simulink model "force_grav"  (R2021a)
settings: Solver=VariableStepAuto  StartTime=0.0  StopTime=100  RelTol=1e-3
values from neighbouring files (symbols this model uses):
  P = [real(P), imag(P)]    [black_pz.m]    (also in black_rlocus.m; black_rlocus_fine.m)
  R = rlocus(sys)    [black_rlocus.m]    (also in black_rlocus_fine.m = rlocus(sys,k))
undefined symbols (not defined in the file or in its folder): A_rocket, alpha_fine, Baro_exp, cm_fine, cm_lookup, Ct_rot, D, drag_lookup, drag_rot_lookup, drag_wave_lookup, g, h_0, I_s, I_x_lookup, I_yz_lookup, L_b, lift_lookup, lift_rot_lookup, m_burn, M_crit, M_fine, m_prop_max, m_wet, N, P_0, Phi, Psi, Q, r_E, S_e, T_b, T_lookup, T_max, T_max_s, t_P, t_S, Theta, U, V, W
libraries: simulink_extras x2
settings Model: Creator=EpEp  LastModifiedBy=EpEp
settings DebuggingCC: UnderSpecifiedDimensionMsg=warning

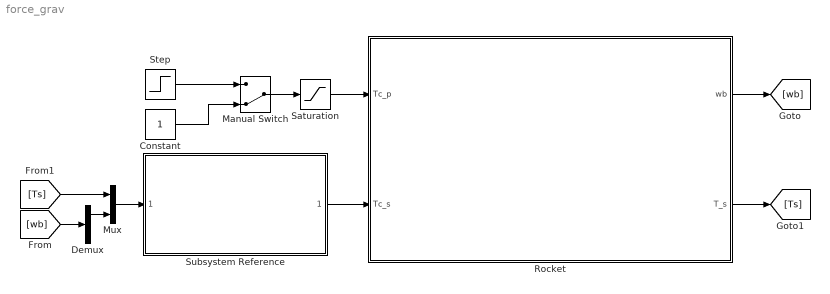
== system force_grav ==
  Constant : Constant
  Demux : Demux  Outputs=3
  Manual Switch : ManualSwitch  CurrentSetting=0
  Mux : Mux  Inputs=2
  Rocket : Subsystem
  Saturation : Saturate  UpperLimit=1  LowerLimit=0.5
  Step : Step  Time=10  Before=1  After=0  SampleTime=0
  Subsystem Reference : Subsystem  ReferencedSubsystem=roll_controller
  wires:
  Constant/1 -> Manual Switch/2
  Step/1 -> Manual Switch/1
  Manual Switch/1 -> Saturation/1
  Saturation/1 -> Rocket/1(Tc_p)
  Mux/1 -> Subsystem Reference/1
  Demux/1 -> Mux/2
  Subsystem Reference/1 -> Rocket/2(Tc_s)
  Rocket/1(wb) -> [wb]
  Rocket/2(T_s) -> [Ts]
  [wb] -> Demux/1
  [Ts] -> Mux/1

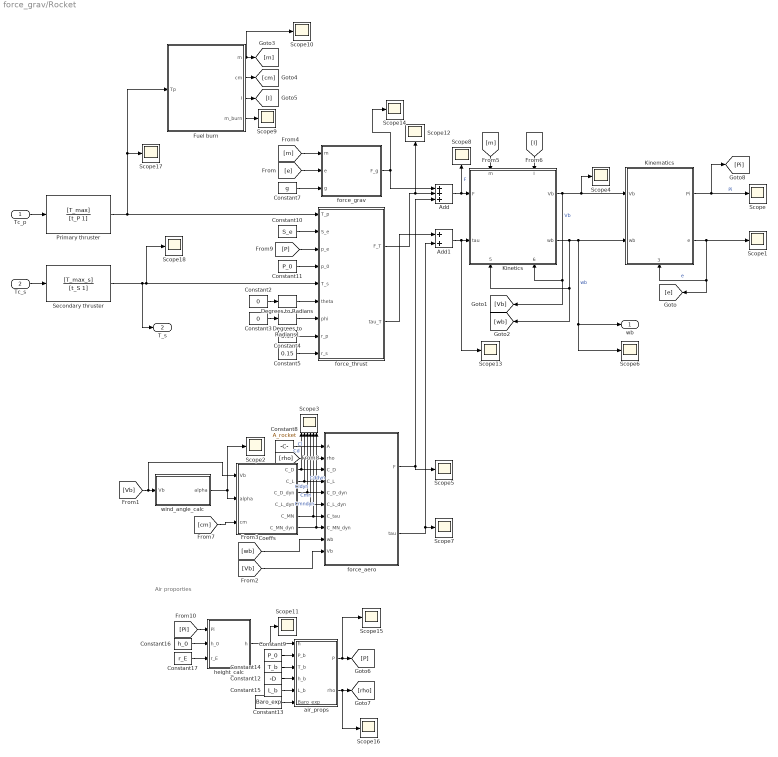
== system force_grav/Rocket ==
  note: Air proporties
  Tc_p : Inport
  Tc_s : Inport  Port=2
  Add : Sum  Inputs=+++
  Add1 : Sum
  Coeffs : Subsystem
  Constant10 : Constant  Value=S_e
  Constant11 : Constant  Value=P_0
  Constant12 : Constant  Value=-D
  Constant13 : Constant  Value=Baro_exp
  Constant14 : Constant  Value=T_b
  Constant15 : Constant  Value=L_b
  Constant16 : Constant  Value=h_0
  Constant17 : Constant  Value=r_E
  Constant2 : Constant  Value=0
  Constant3 : Constant  Value=0
  Constant4 : Constant  Value=0.55
  Constant5 : Constant  Value=0.15
  Constant7 : Constant  Value=g
  Constant8 : Constant  Value=A_rocket
  Constant9 : Constant  Value=P_0
  Degrees to Radians : simulink_extras/Transformations/Degrees to Radians
  Degrees to Radians1 : simulink_extras/Transformations/Degrees to Radians
  Fuel burn : Subsystem
  Kinematics : Subsystem
      settings: PortSchema="{\"entries\":[{\"content\":{\"sides\":[{\"content\":{\"connectorIds\":[\"In1\",\"In2\"]},\"type\":\"ConnectorPlacement.EquallySpacedRectSide\",\"uuid\":\"eae29983-0cae-4ee4-868d-1c50a6f3cfea\"},{\"content\":{\"connectorIds\":[\"Out1\",\"Out2\"],\"side\":\"RIGHT\"},\"type\":\"ConnectorPlacement.EquallySpacedRectSide\",\"uuid\":\"bdc65933-6547-4251-8b39-00a552207d7f\"},{\"content\":{\"connectorIds\":[],\"side\":\"TOP\"},\"type\":\"ConnectorPlacement.EquallySpacedRectSide\",\"uuid\":\"ee33c1e0-7d1f-4e43-84a0-58639e27ac5c\"},{\"content\":{\"connectorIds\":[\"In3\"],\"side\":\"BOTTOM\"},\"type\":\"ConnectorPlacement.EquallySpacedRectSide\",\"uuid\":\"b7ff67e5-658b-4688-8b54-a193f9f6d197\"}]},\"type\":\"ConnectorPlacement.EquallySpacedConnector\",\"uuid\":\"f4d120fb-b3cd-4fc8-b600-b4efda2a2057\"}],\"packageUris\":[\"http://schema.mathworks.com/mf0/Connector/R2020b\"],\"version\":\"1.0\"}"
  Kinetics : Subsystem
      settings: PortSchema="{\"entries\":[{\"content\":{\"sides\":[{\"content\":{\"connectorIds\":[\"In1\",\"In2\"]},\"type\":\"ConnectorPlacement.EquallySpacedRectSide\",\"uuid\":\"44e96cf1-b775-4685-9d80-77fe5197a3b8\"},{\"content\":{\"connectorIds\":[\"Out1\",\"Out2\"],\"side\":\"RIGHT\"},\"type\":\"ConnectorPlacement.EquallySpacedRectSide\",\"uuid\":\"1ce02f86-3039-4a72-8110-79d6c21885aa\"},{\"content\":{\"connectorIds\":[\"In3\",\"In4\"],\"side\":\"TOP\"},\"type\":\"ConnectorPlacement.EquallySpacedRectSide\",\"uuid\":\"c3c088af-4572-4447-8e34-ea7d8079d91e\"},{\"content\":{\"connectorIds\":[\"In5\",\"In6\"],\"side\":\"BOTTOM\"},\"type\":\"ConnectorPlacement.EquallySpacedRectSide\",\"uuid\":\"9c91a776-c86a-41f9-9dfe-00178419c6d9\"}]},\"type\":\"ConnectorPlacement.EquallySpacedConnector\",\"uuid\":\"6fbd1051-4f47-4787-a689-54b5a6d8998f\"}],\"packageUris\":[\"http://schema.mathworks.com/mf0/Connector/R2020b\"],\"version\":\"1.0\"}"
  Primary thruster : TransferFcn  Numerator=[T_max]  Denominator=[t_P 1]
  Scope{,1..2,4..18} (18 alike) : Scope
  Scope3 : Scope  NumInputPorts=6
  Secondary thruster : TransferFcn  Numerator=[T_max_s]  Denominator=[t_S 1]
  air_props : MATLAB Function  TreatAsAtomicUnit=on
  force_aero : MATLAB Function  TreatAsAtomicUnit=on
  force_grav : MATLAB Function  TreatAsAtomicUnit=on
  force_thrust : MATLAB Function  TreatAsAtomicUnit=on
  height_calc : MATLAB Function  TreatAsAtomicUnit=on
  wind_angle_calc : MATLAB Function  TreatAsAtomicUnit=on
  wb : Outport
  T_s : Outport  Port=2
  wires:
  Primary thruster/1 -> Fuel burn/1(Tp), Scope17/1, force_thrust/1(T_p)
  [Vb] -> Coeffs/1(Vb), wind_angle_calc/1(Vb)
  Fuel burn/1(m) -> Scope10/1, [m]
  Kinetics/2(wb) -> [wb], Kinetics/5(5), wb/1, Scope6/1, Kinematics/2(wb)  "wb"
  force_grav/1(F_g) -> Add/1, Scope14/1
  force_aero/2(tau) -> Add1/2, Scope7/1
  Kinematics/1(Pi) -> [Pi], Scope/1  "Pi"
  Kinematics/2(e) -> [e], Kinematics/3(3), Scope1/1  "e"
  Kinetics/1(Vb) -> [Vb], Kinetics/6(6), Scope4/1, Kinematics/1(Vb)  "Vb"
  air_props/2(rho) -> Scope16/1, [rho]
  Coeffs/3(C_D_dyn) -> Scope3/3, force_aero/5(C_D_dyn)  "Cddyn"
  height_calc/1(h) -> Scope11/1, air_props/1(h)
  Constant4/1 -> force_thrust/8(r_p)
  Constant3/1 -> Degrees to Radians1/1
  Add/1 -> Kinetics/1(F), Scope8/1  "F"
  Coeffs/2(C_L) -> Scope3/2, force_aero/4(C_L)  "Cl"
  Degrees to Radians1/1 -> force_thrust/7(phi)
  Add1/1 -> Scope13/1, Kinetics/2(tau)
  Coeffs/4(C_L_dyn) -> Scope3/4, force_aero/6(C_L_dyn)  "Cldyn"
  Coeffs/5(C_MN) -> Scope3/5, force_aero/7(C_tau)  "Cmn"
  Constant9/1 -> air_props/2(P_b)
  force_thrust/2(tau_T) -> Add1/1
  Coeffs/1(C_D) -> Scope3/1, force_aero/3(C_D)  "Cd"
  air_props/1(P) -> Scope15/1, [P]
  [Pi] -> height_calc/1(Pi)
  Constant14/1 -> air_props/3(T_b)
  Coeffs/6(C_MN_dyn) -> Scope3/6, force_aero/8(C_MN_dyn)  "Cmndyn"
  Constant5/1 -> force_thrust/9(r_s)
  Constant7/1 -> force_grav/3(g)
  wind_angle_calc/1(alpha) -> Scope2/1, Coeffs/2(alpha)
  [I] -> Kinetics/4(I)
  Constant16/1 -> height_calc/2(h_0)
  Constant11/1 -> force_thrust/4(p_0)
  Fuel burn/4(m_burn) -> Scope9/1
  [e] -> force_grav/2(e)
  Secondary thruster/1 -> T_s/1, Scope18/1, force_thrust/5(T_s)
  [m] -> force_grav/1(m)
  Constant2/1 -> Degrees to Radians/1
  Constant13/1 -> air_props/6(Baro_exp)
  [m] -> Kinetics/3(m)
  force_aero/1(F) -> Scope5/1, Add/3
  force_thrust/1(F_T) -> Add/2, Scope12/1
  Degrees to Radians/1 -> force_thrust/6(theta)
  [rho] -> force_aero/2(rho)
  [P] -> force_thrust/3(p_e)
  Constant12/1 -> air_props/4(h_b)
  Constant15/1 -> air_props/5(L_b)
  Constant8/1 -> force_aero/1(A)
  [wb] -> force_aero/9(wb)
  Constant10/1 -> force_thrust/2(S_e)
  Constant17/1 -> height_calc/3(r_E)
  Fuel burn/3(I) -> [I]
  [cm] -> Coeffs/3(cm)
  Fuel burn/2(cm) -> [cm]
  [Vb] -> force_aero/10(Vb)
  Tc_p/1 -> Primary thruster/1
  Tc_s/1 -> Secondary thruster/1

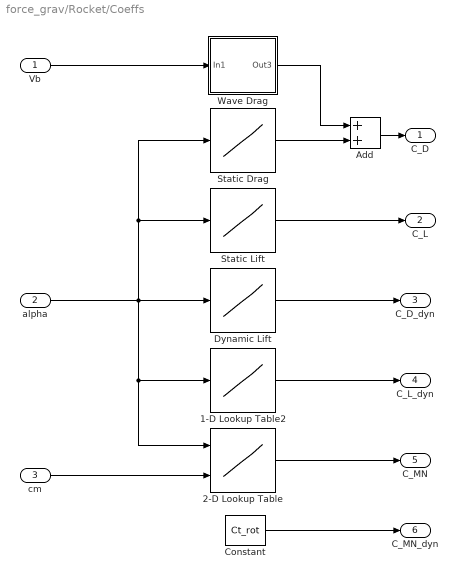
== system force_grav/Rocket/Coeffs ==
  Vb : Inport
  alpha : Inport  Port=2
  cm : Inport  Port=3
  1-D Lookup Table2 : Lookup_n-D  NumberOfTableDimensions=1  BreakpointsForDimension1=alpha_fine  Table=lift_rot_lookup  InternalRulePriority=Speed  RndMeth=Simplest  InputSameDT=on
  2-D Lookup Table : Lookup_n-D  BreakpointsForDimension1=alpha_fine  BreakpointsForDimension2=cm_fine  Table=T_lookup  InternalRulePriority=Speed  RndMeth=Simplest  InputSameDT=on
      settings: InputPortMap=u0,u1
  Add : Sum
  Constant : Constant  Value=Ct_rot
  Dynamic Lift : Lookup_n-D  NumberOfTableDimensions=1  BreakpointsForDimension1=alpha_fine  Table=drag_rot_lookup  InternalRulePriority=Speed  RndMeth=Simplest  InputSameDT=on
  Static Drag : Lookup_n-D  NumberOfTableDimensions=1  BreakpointsForDimension1=alpha_fine  Table=drag_lookup  InternalRulePriority=Speed  RndMeth=Simplest  InputSameDT=on
  Static Lift : Lookup_n-D  NumberOfTableDimensions=1  BreakpointsForDimension1=alpha_fine  Table=lift_lookup  InternalRulePriority=Speed  RndMeth=Simplest  InputSameDT=on
  Wave Drag : Subsystem
  C_D : Outport
  C_L : Outport  Port=2
  C_D_dyn : Outport  Port=3
  C_L_dyn : Outport  Port=4
  C_MN : Outport  Port=5
  C_MN_dyn : Outport  Port=6
  wires:
  alpha/1 -> Static Drag/1, Static Lift/1, 2-D Lookup Table/1, 1-D Lookup Table2/1, Dynamic Lift/1
  cm/1 -> 2-D Lookup Table/2
  Static Lift/1 -> C_L/1
  Dynamic Lift/1 -> C_D_dyn/1
  1-D Lookup Table2/1 -> C_L_dyn/1
  2-D Lookup Table/1 -> C_MN/1
  Constant/1 -> C_MN_dyn/1
  Static Drag/1 -> Add/2
  Vb/1 -> Wave Drag/1(In1)
  Wave Drag/1(Out3) -> Add/1
  Add/1 -> C_D/1

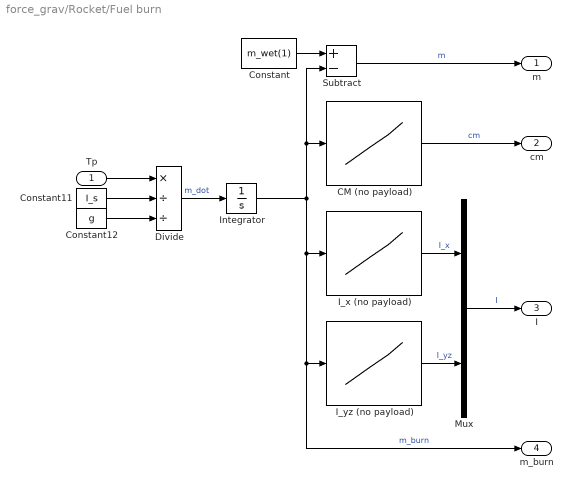
== system force_grav/Rocket/Fuel burn ==
  Tp : Inport
  CM (no payload) : Lookup_n-D  NumberOfTableDimensions=1  BreakpointsForDimension1=[0,m_prop_max*2]  Table=cm_lookup  InternalRulePriority=Speed  RndMeth=Simplest  InputSameDT=on
  Constant : Constant  Value=m_wet(1)
  Constant11 : Constant  Value=I_s
  Constant12 : Constant  Value=g
  Divide : Product  Inputs=*//
  I_x (no payload) : Lookup_n-D  NumberOfTableDimensions=1  BreakpointsForDimension1=[0,m_prop_max*2]  Table=I_x_lookup  InternalRulePriority=Speed  RndMeth=Simplest  InputSameDT=on
  I_yz (no payload) : Lookup_n-D  NumberOfTableDimensions=1  BreakpointsForDimension1=m_burn*2  Table=I_yz_lookup  InternalRulePriority=Speed  RndMeth=Simplest  InputSameDT=on
  Integrator : Integrator
  Mux : Mux  Inputs=2
  Subtract : Sum  Inputs=+-
  m : Outport
  cm : Outport  Port=2
  I : Outport  Port=3
  m_burn : Outport  Port=4
  wires:
  Divide/1 -> Integrator/1  "m_dot"
  Constant11/1 -> Divide/2
  Integrator/1 -> m_burn/1, I_yz (no payload)/1, I_x (no payload)/1, Subtract/2, CM (no payload)/1  "m_burn"
  Tp/1 -> Divide/1
  Constant/1 -> Subtract/1
  Subtract/1 -> m/1  "m"
  CM (no payload)/1 -> cm/1  "cm"
  I_x (no payload)/1 -> Mux/1  "I_x"
  I_yz (no payload)/1 -> Mux/2  "I_yz"
  Mux/1 -> I/1  "I"
  Constant12/1 -> Divide/3

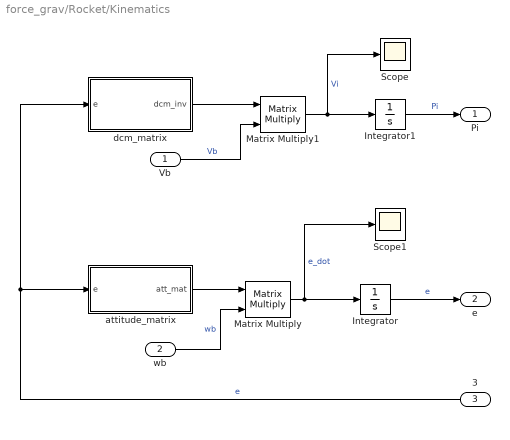
== system force_grav/Rocket/Kinematics ==
  Vb : Inport
  wb : Inport  Port=2
  3 : Inport  Port=3
  Integrator : Integrator  InitialCondition=[Phi;Theta;Psi]
  Integrator1 : Integrator  InitialCondition=[N;E;D]
  Matrix Multiply : Product  Multiplication=Matrix(*)
  Matrix Multiply1 : Product  Multiplication=Matrix(*)
  Scope : Scope
  Scope1 : Scope
  attitude_matrix : MATLAB Function  TreatAsAtomicUnit=on
  dcm_matrix : MATLAB Function  TreatAsAtomicUnit=on
  Pi : Outport
  e : Outport  Port=2
  wires:
  attitude_matrix/1(att_mat) -> Matrix Multiply/1
  wb/1 -> Matrix Multiply/2  "wb"
  Matrix Multiply/1 -> Scope1/1, Integrator/1  "e_dot"
  Integrator/1 -> e/1  "e"
  dcm_matrix/1(dcm_inv) -> Matrix Multiply1/1
  Vb/1 -> Matrix Multiply1/2  "Vb"
  Matrix Multiply1/1 -> Scope/1, Integrator1/1  "Vi"
  Integrator1/1 -> Pi/1  "Pi"
  3/1 -> dcm_matrix/1(e), attitude_matrix/1(e)  "e"

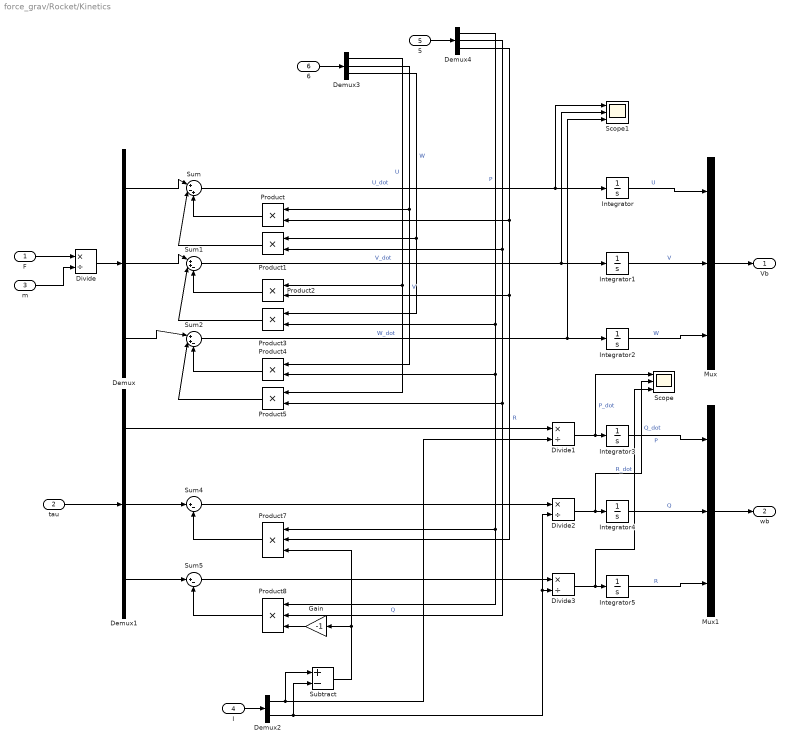
== system force_grav/Rocket/Kinetics ==
  F : Inport  PortDimensions=[3,1]
  tau : Inport  Port=2  PortDimensions=[3,1]
  m : Inport  Port=3
  I : Inport  Port=4
  5 : Inport  Port=5
  6 : Inport  Port=6
  Demux{,1,3..4} (4 alike) : Demux  Outputs=3
  Demux2 : Demux  Outputs=2
  Divide{,1..3} (4 alike) : Product  Inputs=*/
  Gain : Gain  Gain=-1
  Integrator : Integrator  InitialCondition=U
  Integrator1 : Integrator  InitialCondition=V
  Integrator2 : Integrator  InitialCondition=W
  Integrator3 : Integrator  InitialCondition=P
  Integrator4 : Integrator  InitialCondition=Q
  Integrator5 : Integrator  InitialCondition=R
  Mux : Mux  Inputs=3
  Mux1 : Mux  Inputs=3
  Product{,1..5} (6 alike) : Product
  Product7 : Product  Inputs=3
  Product8 : Product  Inputs=3
  Scope : Scope  NumInputPorts=3
  Scope1 : Scope  NumInputPorts=3
  Subtract : Sum  Inputs=+-
  Sum : Sum  Inputs=|+-+
  Sum1 : Sum  Inputs=|++-
  Sum2 : Sum  Inputs=|++-
  Sum4 : Sum  Inputs=|+-
  Sum5 : Sum  Inputs=|+-
  Vb : Outport  PortDimensions=[3,1]
  wb : Outport  Port=2  PortDimensions=[3,1]
  wires:
  Demux/1 -> Sum/1
  Demux1/3 -> Sum5/1
  Demux/2 -> Sum1/1
  Demux/3 -> Sum2/1
  Demux1/2 -> Sum4/1
  Product1/1 -> Sum/2
  Product/1 -> Sum/3
  Product3/1 -> Sum1/2
  Product2/1 -> Sum1/3
  Product4/1 -> Sum2/3
  Product5/1 -> Sum2/2
  F/1 -> Divide/1
  Divide/1 -> Demux/1
  m/1 -> Divide/2
  tau/1 -> Demux1/1
  Product7/1 -> Sum4/2
  Product8/1 -> Sum5/2
  Demux1/1 -> Divide1/1
  Divide1/1 -> Scope/1, Integrator3/1  "P_dot"
  Sum/1 -> Scope1/1, Integrator/1  "U_dot"
  Sum1/1 -> Scope1/2, Integrator1/1  "V_dot"
  Sum2/1 -> Scope1/3, Integrator2/1  "W_dot"
  I/1 -> Demux2/1
  Demux2/1 -> Divide1/2, Subtract/1
  Divide2/1 -> Scope/2, Integrator4/1  "Q_dot"
  Divide3/1 -> Scope/3, Integrator5/1  "R_dot"
  Sum5/1 -> Divide3/1
  Sum4/1 -> Divide2/1
  Demux2/2 -> Divide3/2, Divide2/2, Subtract/2
  Subtract/1 -> Product7/3, Gain/1
  Gain/1 -> Product8/3
  6/1 -> Demux3/1
  5/1 -> Demux4/1
  Demux3/2 -> Product4/1, Product/1  "V"
  Demux4/3 -> Product7/2, Product2/2, Product/2  "R"
  Demux3/3 -> Product3/1, Product1/1  "W"
  Demux4/1 -> Product3/2, Product8/1, Product7/1, Product4/2  "P"
  Demux3/1 -> Product5/1, Product2/1  "U"
  Demux4/2 -> Product1/2, Product5/2, Product8/2  "Q"
  Integrator/1 -> Mux/1  "U"
  Integrator2/1 -> Mux/3  "W"
  Integrator1/1 -> Mux/2  "V"
  Mux/1 -> Vb/1
  Integrator5/1 -> Mux1/3  "R"
  Integrator4/1 -> Mux1/2  "Q"
  Integrator3/1 -> Mux1/1  "P"
  Mux1/1 -> wb/1

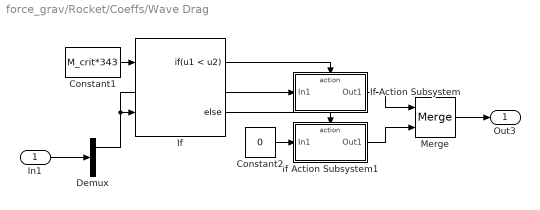
== system force_grav/Rocket/Coeffs/Wave Drag ==
  In1 : Inport
  Constant1 : Constant  Value=M_crit*343
  Constant2 : Constant  Value=0
  Demux : Demux  Outputs=3
  If : If  NumInputs=2  IfExpression=u1 < u2
  If Action Subsystem : Subsystem  TreatAsAtomicUnit=on
  If Action Subsystem1 : Subsystem  TreatAsAtomicUnit=on
  Merge : Merge
  Out3 : Outport
  wires:
  Merge/1 -> Out3/1
  If/2 -> If Action Subsystem1/Action
  Demux/1 -> If/2, If Action Subsystem/1(In1)
  If Action Subsystem1/1(Out1) -> Merge/2
  Constant1/1 -> If/1
  If Action Subsystem/1(Out1) -> Merge/1
  If/1 -> If Action Subsystem/Action
  Constant2/1 -> If Action Subsystem1/1(In1)
  In1/1 -> Demux/1

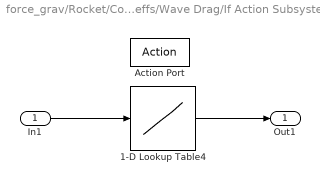
== system force_grav/Rocket/Coeffs/Wave Drag/If Action Subsystem ==
  In1 : Inport
  Action Port : ActionPort  ActionPortLabel=if(u1 < u2)
  1-D Lookup Table4 : Lookup_n-D  NumberOfTableDimensions=1  BreakpointsForDimension1=M_fine*343  Table=drag_wave_lookup  InternalRulePriority=Speed  RndMeth=Simplest  InputSameDT=on
  Out1 : Outport
  wires:
  In1/1 -> 1-D Lookup Table4/1
  1-D Lookup Table4/1 -> Out1/1

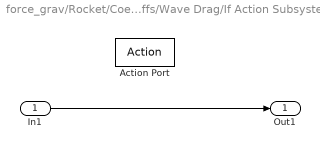
== system force_grav/Rocket/Coeffs/Wave Drag/If Action Subsystem1 ==
  In1 : Inport
  Action Port : ActionPort  ActionPortLabel=else
  Out1 : Outport
  wires:
  In1/1 -> Out1/1

== matlab function force_grav/Rocket/force_thrust ==
  data: T_p input; S_e input; p_e input; p_0 input; F_T output; T_s input; theta input; phi input; r_p input; r_s input; tau_T output
function [F_T, tau_T] = fcn(T_p,S_e,p_e,p_0, T_s, theta, phi, r_p, r_s)
    if T_p ~= 0
        T_p = T_p + S_e*(p_0-p_e);
    end
    F_mat = [cos(theta); 
             sin(theta)*cos(phi); 
             sin(theta)*cos(pi/2-phi)];
    F_T = F_mat*T_p;
    tau_T = [T_s*r_s; 
             F_T(3)*r_p; 
             F_T(2)*r_p];

== matlab function force_grav/Rocket/force_grav ==
  data: m input; F_g output; e input; g input
function F_g = fcn(m,e,g)
    Phi = e(1);
    Theta = e(2);
    Psi = e(3);
    grav_mat = [-cos(Psi)*cos(Theta);
                -cos(Psi)*sin(Theta)*sin(Phi) + sin(Psi)*cos(Phi);
                -cos(Psi)*sin(Theta)*cos(Phi) + sin(Psi)*sin(Phi)];
    F_g = grav_mat*m*g;

== matlab function force_grav/Rocket/Kinematics/attitude_matrix ==
  data: att_mat output; e input
function att_mat = fcn(e)
    Phi = e(1);
    Theta = e(2);
    att_mat = [1    , sin(Phi)*tan(Theta)   , cos(Phi)*tan(Theta)   ;
               0    , cos(Phi)              , -sin(Phi)             ;
               0    , sin(Phi)*sec(Theta)   , cos(Phi)*sec(Theta)   ;];

== matlab function force_grav/Rocket/Kinematics/dcm_matrix ==
  data: e input; dcm_inv output
function dcm_inv = fcn(e)
    Phi = e(1);
    Theta = e(2);
    Psi = e(3);
    
    dcm_inv = [-sin(Theta)          , cos(Theta)*sin(Phi)                               , cos(Theta)*cos(Phi)                               ;
                sin(Psi)*cos(Theta) , sin(Psi)*sin(Theta)*sin(Phi) + cos(Psi)*cos(Phi)  , sin(Psi)*sin(Theta)*cos(Phi) - cos(Psi)*sin(Phi)  ;
               -cos(Psi)*cos(Theta) , -cos(Psi)*sin(Theta)*sin(Phi) + sin(Psi)*cos(Phi) , -cos(Psi)*sin(Theta)*cos(Phi) - sin(Psi)*sin(Phi) ;];

== matlab function force_grav/Rocket/force_aero ==
  data: A input; rho input; C_D input; F output; tau output; C_L input; C_D_dyn input; C_L_dyn input; C_tau input; C_MN_dyn input; wb input; Vb input
function [F,tau] = fcn(A,rho,C_D,C_L,C_D_dyn,C_L_dyn,C_tau,C_MN_dyn,wb,Vb)
    Vb_norm_sqr = Vb'*Vb;
    % Get unit velocity vector
    if Vb_norm_sqr ~= 0
        Vb_unit = Vb/sqrt(Vb_norm_sqr);
    else
        Vb_unit = Vb;
    end
    
    % Get unit force vectors
    Drag_vec = -Vb_unit;
    Torque_vec = cross(Vb_unit,[1;0;0]);
    Lift_vec = cross(Torque_vec,Vb_unit);
    
    C_XYZ = Drag_vec*C_D + Lift_vec*C_L;
    C_LMN = Torque_vec*C_tau;
    
    F = 0.5*rho*A*Vb_norm_sqr*C_XYZ;
    tau = 0.5*rho*A*Vb_norm_sqr*C_LMN;

== matlab function force_grav/Rocket/wind_angle_calc ==
  data: Vb input; alpha output
function alpha  = fcn(Vb)
    Vb_norm = sqrt(Vb'*Vb);
    if Vb_norm ~= 0
        alpha = acos(dot(Vb/Vb_norm,[1;0;0]));
    else
        alpha = 0;
    end

== matlab function force_grav/Rocket/air_props ==
  data: h input; P output; rho output; P_b input; T_b input; h_b input; L_b input; Baro_exp input
function [P,rho] = fcn(h,P_b,T_b,h_b,L_b,Baro_exp)
    T = T_b+(h-h_b)*L_b;
    P = P_b*(T/T_b)^Baro_exp;
    rho = (P*0.02897)/(8.3145*T);

== matlab function force_grav/Rocket/height_calc ==
  data: Pi input; h output; h_0 input; r_E input
function h = fcn(Pi,h_0,r_E)
    h = sqrt(Pi(1)^2+Pi(2)^2+(r_E+h_0-Pi(3))^2)-r_E;
